simulink model "Homework4_P3"  (R2023b)
settings: Solver=VariableStepAuto  StartTime=0.0  StopTime=10  FixedStep=0.002  RelTol=1e-3  EnableMultiTasking=on
libraries: simulink x3
settings Model: ExtModeTrigDuration=10000  Creator=jtmil  LastModifiedBy=jtmil
settings SolverCC: AlgebraicLoopSolver=TrustRegion  PositivePriorityOrder=on
settings DataIOCC: ReturnWorkspaceOutputs=off
settings OptimizationCC: LifeSpan=inf
settings DebuggingCC: UnconnectedInputMsg=warning  UnconnectedOutputMsg=warning  UnconnectedLineMsg=warning  ArithmeticOperatorsInVariantConditions=warning
settings ModelReferenceCC: EnableRefExpFcnMdlSchedulingChecks=on
settings SFSimCC: SimUseLocalCustomCode=off  CustomCodeUndefinedFunction=UseInterfaceOnly
settings RTWCC: Description=QUARC Win64 Target  SystemTargetFile=quarc_win64.tlc  TemplateMakefile=quarc_default_tmf  RTWUseLocalCustomCode=off
settings CodeAppCC: StateflowObjectComments=on
settings STFCustomTargetCC: TargetPreCompLibLocation=C:\PROGRA~3\QUARC\lib\2016a\win64\release  ConcurrentExecutionCompliant=on  GRTInterface=on  SystemTargetFile=quarc_win64.tlc
settings GRTTargetCC: TargetPreCompLibLocation=C:\PROGRA~3\QUARC\lib\2016a\win64\release  ParMdlRefBuildCompliant=off  CompOptLevelCompliant=off  CombineOutputUpdateFcns=off  MatFileLogging=off  CPPClassGenCompliant=off  GRTInterface=on  UseToolchainInfoCompliant=off  ExtMode=on  ExtModeMexFile=quarc_comm
settings ConfigComp: CovMetricSettings=dswe

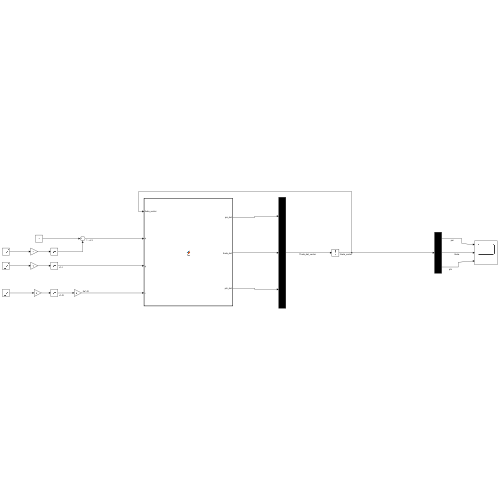
[thumbnail: Simulink's stored preview of the top-level diagram]
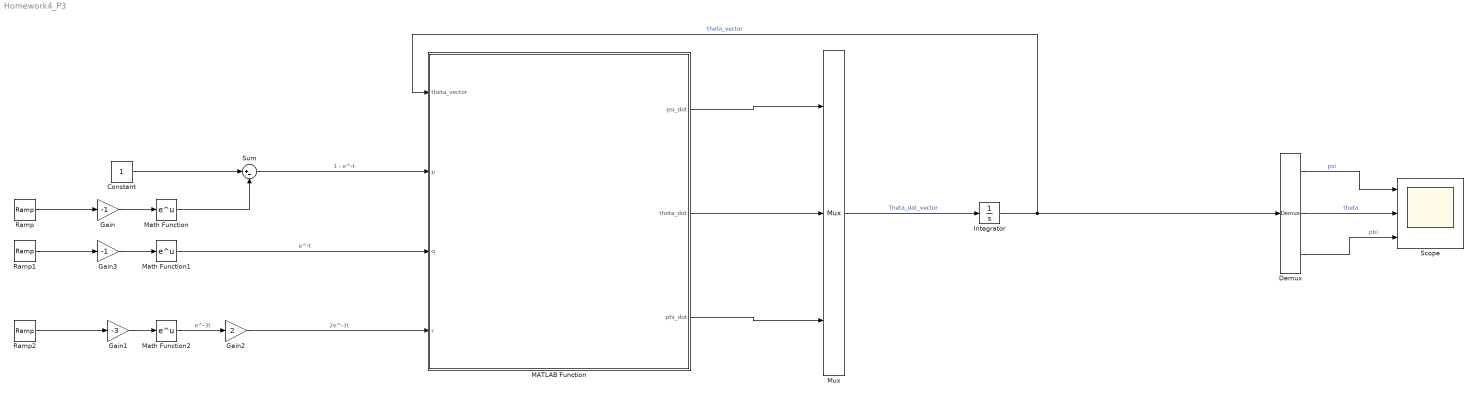
== system Homework4_P3 ==
  Constant : Constant
  Demux : Demux  Outputs=3
  Gain : Gain  Gain=-1
  Gain1 : Gain  Gain=-3
  Gain2 : Gain  Gain=2
  Gain3 : Gain  Gain=-1
  Integrator : Integrator  InitialCondition=[0;45;0]
  MATLAB Function : MATLAB Function  TreatAsAtomicUnit=on
  Math Function : Math
  Math Function1 : Math
  Math Function2 : Math
  Mux : Mux  Inputs=3
  Ramp : simulink/Sources/Ramp  slope=1  start=0  InitialOutput=0
  Ramp1 : simulink/Sources/Ramp  slope=1  start=0  InitialOutput=0
  Ramp2 : simulink/Sources/Ramp  slope=1  start=0  InitialOutput=0
  Scope : Scope  NumInputPorts=3
  Sum : Sum  Inputs=|+-
  wires:
  Math Function/1 -> Sum/2
  Constant/1 -> Sum/1
  Math Function2/1 -> Gain2/1  "e^-3t"
  Gain1/1 -> Math Function2/1
  Gain2/1 -> MATLAB Function/4(r)  "2e^-3t"
  Math Function1/1 -> MATLAB Function/3(q)  "e^-t"
  Sum/1 -> MATLAB Function/2(p)  "1 - e^-t"
  MATLAB Function/1(psi_dot) -> Mux/1
  MATLAB Function/2(theta_dot) -> Mux/2
  MATLAB Function/3(phi_dot) -> Mux/3
  Mux/1 -> Integrator/1  "Theta_dat_vector"
  Integrator/1 -> Demux/1, MATLAB Function/1(theta_vector)  "theta_vector"
  Demux/2 -> Scope/2  "theta"
  Demux/1 -> Scope/1  "psi"
  Demux/3 -> Scope/3  "phi"
  Gain/1 -> Math Function/1
  Gain3/1 -> Math Function1/1
  Ramp/1 -> Gain/1
  Ramp1/1 -> Gain3/1
  Ramp2/1 -> Gain1/1

== matlab function Homework4_P3/MATLAB Function ==
  data: theta_vector input; p input; psi_dot output; q input; r input; theta_dot output; phi_dot output
function [psi_dot, theta_dot, phi_dot] = fcn(theta_vector, p, q, r)

w_B = [p; q; r];

psi = theta_vector(1);
theta = theta_vector(2);
phi = theta_vector(3);

B_inv = (1/cosd(theta))*[0, sind(phi), cosd(phi); 
         0, cosd(phi)*cosd(theta), -sind(phi)*cosd(theta); 
         cosd(theta), sind(phi)*sind(theta), cosd(phi)*sind(theta)];

theta_dot_vector = B_inv * w_B; 

psi_dot = theta_dot_vector(1); 
theta_dot = theta_dot_vector(2);
phi_dot = theta_dot_vector(3);

end
